simulink model "FTBO_Eq_diff_Vm_oc"  (R2021b)
settings: Solver=VariableStepAuto  StartTime=0.0  StopTime=10  RelTol=1e-3
undefined symbols (not defined in the file): Eq_diff_coeff_oc, Eq_diff_coeff_Vm, kbb
settings Model: Creator=levm1106  LastModifiedBy=sama1402

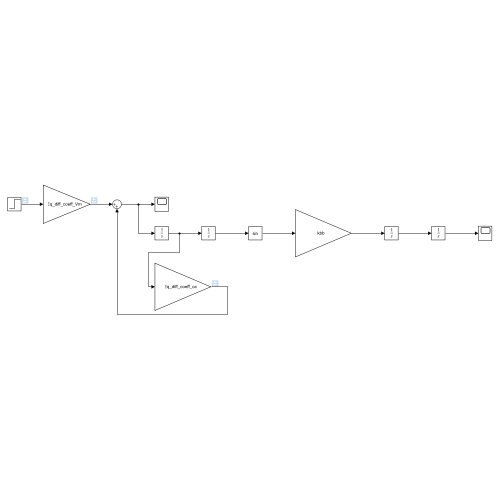
[thumbnail: Simulink's stored preview of the top-level diagram]
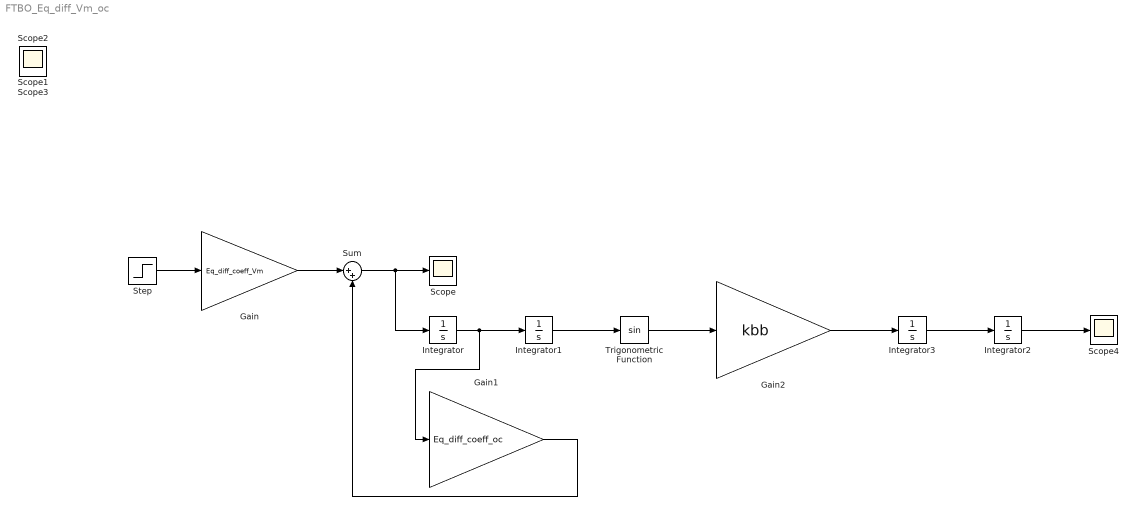
== system FTBO_Eq_diff_Vm_oc ==
  Gain : Gain  Gain=Eq_diff_coeff_Vm
  Gain1 : Gain  Gain=Eq_diff_coeff_oc
  Gain2 : Gain  Gain=kbb
  Integrator{,1..3} (4 alike) : Integrator
  Scope{,1..4} (5 alike) : Scope
  Step : Step  Time=0  Before=1  SampleTime=0
  Sum : Sum  Inputs=|++
  Trigonometric Function : Trigonometry
  wires:
  Step/1 -> Gain/1
  Gain/1 -> Sum/1
  Sum/1 -> Integrator/1, Scope/1
  Integrator/1 -> Integrator1/1, Gain1/1
  Gain1/1 -> Sum/2
  Integrator1/1 -> Trigonometric Function/1
  Trigonometric Function/1 -> Gain2/1
  Gain2/1 -> Integrator3/1
  Integrator3/1 -> Integrator2/1
  Integrator2/1 -> Scope4/1
